simulink model "FlightSim"  (R2023a)
settings: Solver=VariableStepAuto  StartTime=0.0  StopTime=10.0  RelTol=1e-3
model workspace (MAT data in the model file):
  polyCoefficient = [1 1 1]
values from neighbouring files (symbols this model uses):
  mass = 4    [FlightSimSetup.m]
settings Model: Creator=ericyang  LastModifiedBy=ericyang
settings DataIOCC: ExternalInput=[t,u]

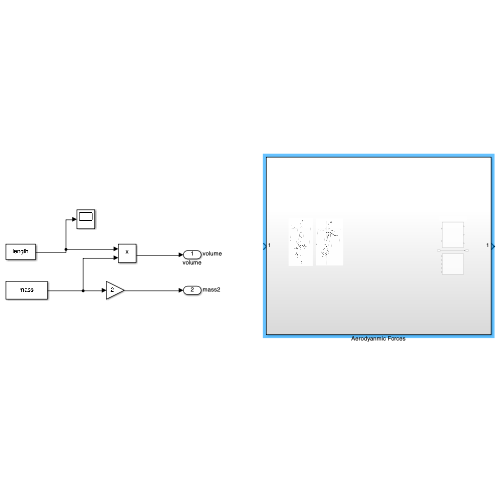
[thumbnail: Simulink's stored preview of the top-level diagram]
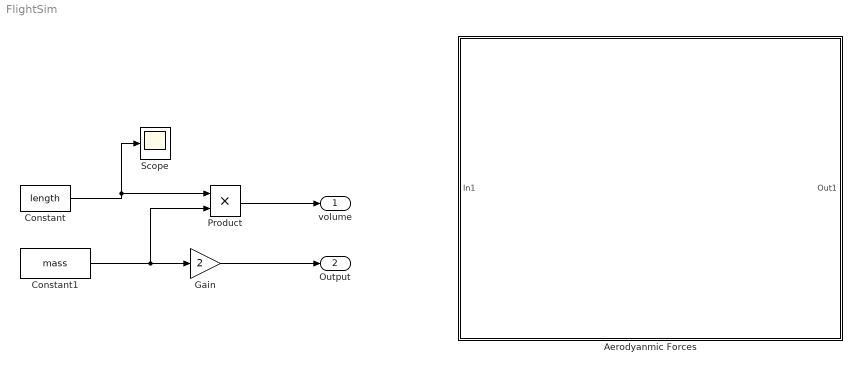
== system FlightSim ==
  Aerodyanmic Forces : Subsystem
  Constant : Constant  Value=length
  Constant1 : Constant  Value=mass
  Gain : Gain  Gain=2
  Product : Product
  Scope : Scope
  volume : Outport  SignalName=volume
  Output : Outport  Port=2  SignalName=mass2
  wires:
  Constant/1 -> Product/1, Scope/1
  Constant1/1 -> Gain/1, Product/2
  Product/1 -> volume/1
  Gain/1 -> Output/1

== system FlightSim/Aerodyanmic Forces ==
  note: calculates the total N and Center of Pressure shown in the diagram based on contriutions from each rocket part, and from those also calculates pitch
  In1 : Inport
  Canard Roll Calc : Subsystem
  Normal Force and Pitch Moment Calc : Subsystem
  Out1 : Outport
  wires:
  In1/1 -> Out1/1

== system FlightSim/Aerodyanmic Forces/Canard Roll Calc ==
  radialMACPosition : Inport
  bodyDiameter : Inport  Port=2
  CNa : Inport  Port=3
  numFins : Inport  Port=4
  rollAngle : Inport  Port=5
  RollForcingCoefficient : Subsystem
  RollForcingCoefficient1 : Subsystem
  wires:
  radialMACPosition/1 -> RollForcingCoefficient/1(radialMACPosition)
  bodyDiameter/1 -> RollForcingCoefficient/2(bodyDiameter)
  CNa/1 -> RollForcingCoefficient/3(CNa)
  numFins/1 -> RollForcingCoefficient/4(numFins)
  rollAngle/1 -> RollForcingCoefficient/5(rollAngle)

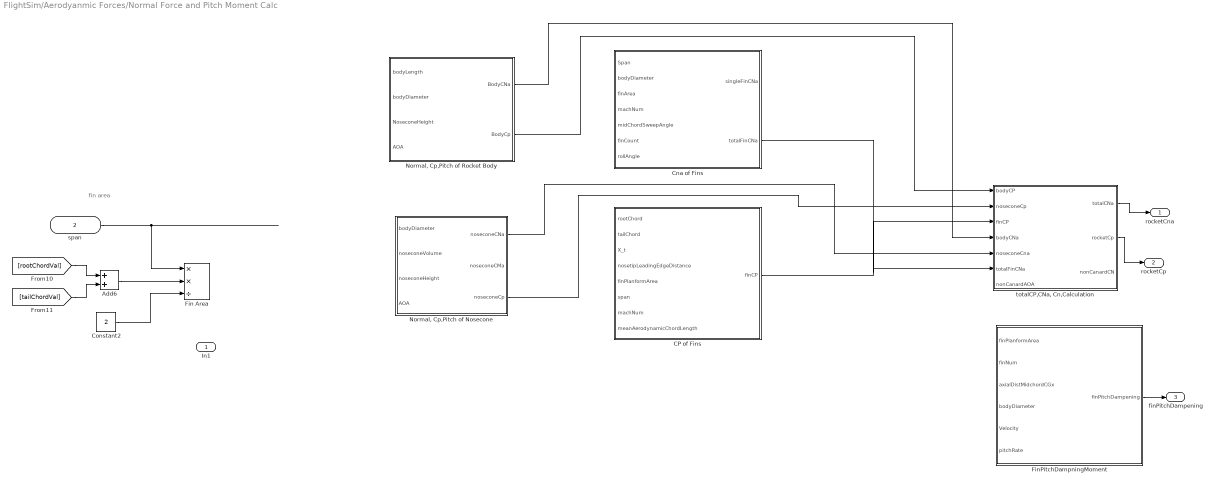
== system FlightSim/Aerodyanmic Forces/Normal Force and Pitch Moment Calc ==
  note: fin area
  In1 : Inport
  span : Inport  Port=2
  Add6 : Sum
  CP of Fins : Subsystem
  Cna of Fins : Subsystem
  Constant2 : Constant  Value=2
  Fin Area : Product  Inputs=**/
  FinPitchDampningMoment : Subsystem
  "Normal, Cp,Pitch of Nosecone" : Subsystem
  "Normal, Cp,Pitch of Rocket Body" : Subsystem
  "totalCP,CNa, Cn,Calculation" : Subsystem
  rocketCna : Outport
  rocketCp : Outport  Port=2
  finPitchDampening : Outport  Port=3
  wires:
  Add6/1 -> Fin Area/2
  span/1 -> Fin Area/1
  [tailChordVal] -> Add6/2
  [rootChordVal] -> Add6/1
  Constant2/1 -> Fin Area/3
  "Normal, Cp,Pitch of Rocket Body"/1(BodyCNa) -> "totalCP,CNa, Cn,Calculation"/4(bodyCNa)
  "Normal, Cp,Pitch of Rocket Body"/2(BodyCp) -> "totalCP,CNa, Cn,Calculation"/1(bodyCP)
  Cna of Fins/2(totalFinCNa) -> "totalCP,CNa, Cn,Calculation"/6(totalFinCNa)
  CP of Fins/1(finCP) -> "totalCP,CNa, Cn,Calculation"/3(finCP)
  "Normal, Cp,Pitch of Nosecone"/3(noseconeCp) -> "totalCP,CNa, Cn,Calculation"/2(noseconeCp)
  "Normal, Cp,Pitch of Nosecone"/1(noseconeCNa) -> "totalCP,CNa, Cn,Calculation"/5(noseconeCna)
  "totalCP,CNa, Cn,Calculation"/1(totalCNa) -> rocketCna/1
  "totalCP,CNa, Cn,Calculation"/2(rocketCp) -> rocketCp/1
  FinPitchDampningMoment/1(finPitchDampening) -> finPitchDampening/1

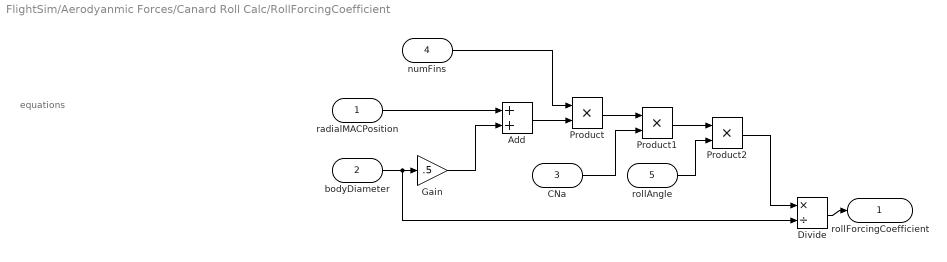
== system FlightSim/Aerodyanmic Forces/Canard Roll Calc/RollForcingCoefficient ==
  note: equations
  radialMACPosition : Inport
  bodyDiameter : Inport  Port=2
  CNa : Inport  Port=3
  numFins : Inport  Port=4
  rollAngle : Inport  Port=5
  Add : Sum
  Divide : Product  Inputs=*/
  Gain : Gain  Gain=.5
  Product : Product
  Product1 : Product
  Product2 : Product
  rollForcingCoefficient : Outport
  wires:
  radialMACPosition/1 -> Add/1
  bodyDiameter/1 -> Divide/2, Gain/1
  rollAngle/1 -> Product2/2
  CNa/1 -> Product1/2
  Divide/1 -> rollForcingCoefficient/1
  Product2/1 -> Divide/1
  Product1/1 -> Product2/1
  Gain/1 -> Add/2
  Product/1 -> Product1/1
  numFins/1 -> Product/1
  Add/1 -> Product/2

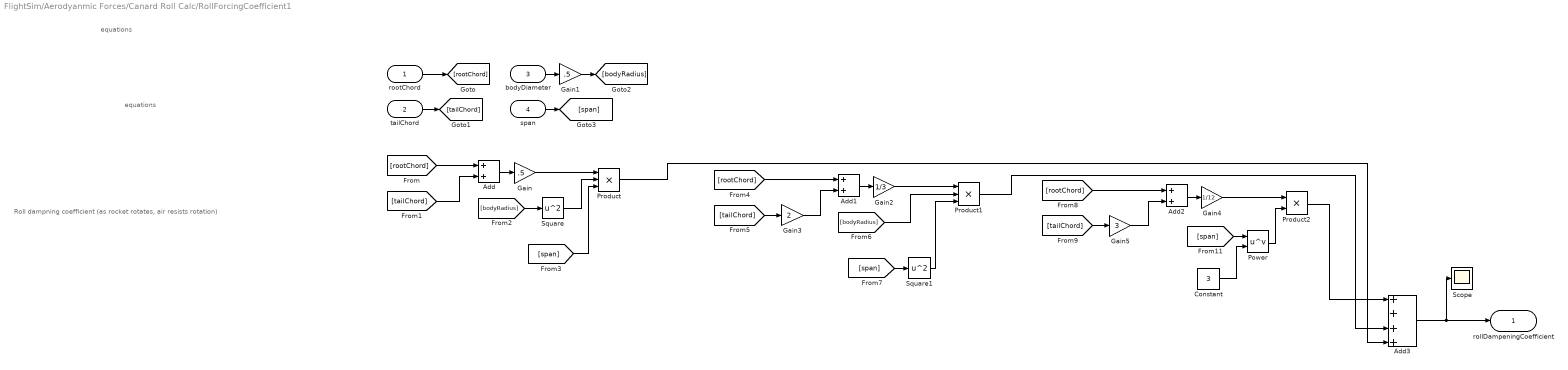
== system FlightSim/Aerodyanmic Forces/Canard Roll Calc/RollForcingCoefficient1 ==
  note: Roll dampning coefficient (as rocket rotates, air resists rotation)
  note: equations
  note: equations
  rootChord : Inport
  tailChord : Inport  Port=2
  bodyDiameter : Inport  Port=3
  span : Inport  Port=4
  Add : Sum
  Add1 : Sum
  Add2 : Sum
  Add3 : Sum  Inputs=++++
  Constant : Constant  Value=3
  Gain : Gain  Gain=.5
  Gain1 : Gain  Gain=.5
  Gain2 : Gain  Gain=1/3
  Gain3 : Gain  Gain=2
  Gain4 : Gain  Gain=1/12
  Gain5 : Gain  Gain=3
  Power : Math  Operator=pow
  Product : Product  Inputs=3
  Product1 : Product  Inputs=3
  Product2 : Product
  Scope : Scope
  Square : Math  Operator=square
  Square1 : Math  Operator=square
  rollDampeningCoefficient : Outport
  wires:
  Add/1 -> Gain/1
  rootChord/1 -> [rootChord]
  tailChord/1 -> [tailChord]
  bodyDiameter/1 -> Gain1/1
  span/1 -> [span]
  [rootChord] -> Add/1
  [tailChord] -> Add/2
  Gain/1 -> Product/1
  Gain1/1 -> [bodyRadius]
  [bodyRadius] -> Square/1
  Square/1 -> Product/2
  [span] -> Product/3
  [tailChord] -> Gain3/1
  [rootChord] -> Add1/1
  Add1/1 -> Gain2/1
  Gain2/1 -> Product1/1
  Gain3/1 -> Add1/2
  [span] -> Square1/1
  Square1/1 -> Product1/3
  [bodyRadius] -> Product1/2
  [span] -> Power/1
  [tailChord] -> Gain5/1
  Gain5/1 -> Add2/2
  [rootChord] -> Add2/1
  Add2/1 -> Gain4/1
  Gain4/1 -> Product2/1
  Constant/1 -> Power/2
  Power/1 -> Product2/2
  Product2/1 -> Add3/1
  Product1/1 -> Add3/3
  Product/1 -> Add3/4
  Add3/1 -> Scope/1, rollDampeningCoefficient/1

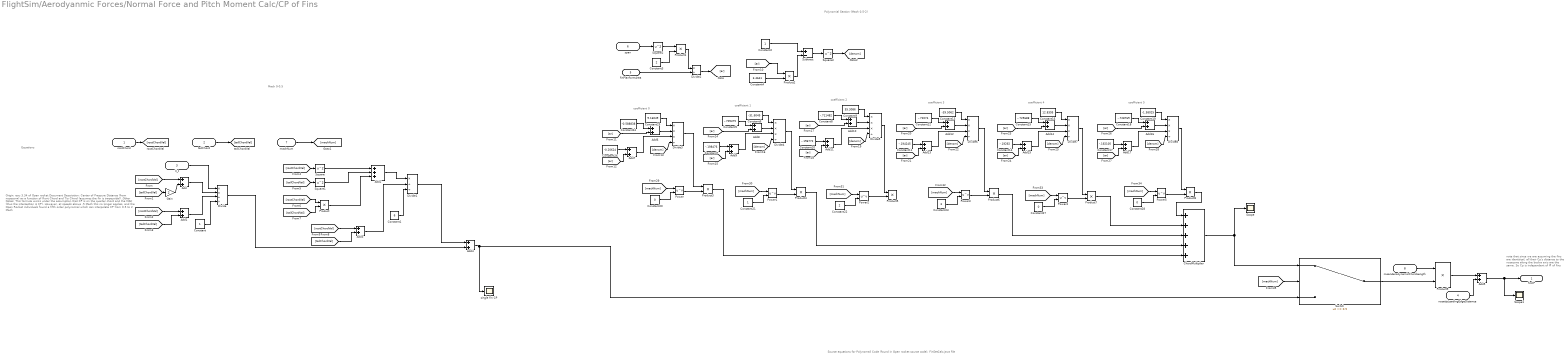
== system FlightSim/Aerodyanmic Forces/Normal Force and Pitch Moment Calc/CP of Fins ==
  note: note that since we are assuming the fins are identitical, all their Cp's distance to the nosecone along the bodya axis are the same. So Cp is independent of # of fins
  note: Mach 0-0.5
  note: Source equations for Polynomail Code (found in Open rocket source code), FinSetCalc.java file
  note: Polynomial Section (Mach 0.5-2)
  note: coefficient 0
  note: Equations
  note: Origin: equ 3.34  of Open rocket Document
      |
      | Description: Center of Pressure Distance (from nosecone)
      | as a function of Root Chord and Tip Chord (assumes the fin is trapezoidal).
      |
      | Other Notes: This formula works under the assumption that CP is on the quarter chord
      | and the MAC (thus the intersection is CP). However, at speeds above .5 Mach this no longer applies, and the Open Rocket individuals found a fifth order polynomial which can interpolate CP from 0.5 to 2 Mach
  note: coefficient 1
  note: coefficient 2
  note: coefficient 3
  note: coefficient 4
  note: coefficient 5
  rootChord : Inport
  tailChord : Inport  Port=2
  X_t : Inport  Port=3
  nosetipLeadingEdgeDistance : Inport  Port=4
  finPlanformArea : Inport  Port=5
  span : Inport  Port=6
  machNum : Inport  Port=7
  meanAerodynamicChordLength : Inport  Port=8
  Add{,1,3..17} (17 alike) : Sum
  Add2 : Sum  Inputs=+++
  ChordMultiplier : Sum  Inputs=+++++
  Constant : Constant
  Constant1 : Constant  Value=6
  Constant10 : Constant  Value=-.196772
  Constant11 : Constant  Value=-.194245
  Constant12 : Constant  Value=-.72074
  Constant13 : Constant  Value=-39.5062
  Constant14 : Constant  Value=-.19292
  Constant15 : Constant  Value=-.725688
  Constant16 : Constant  Value=12.8395
  Constant17 : Constant  Value=-.192105
  Constant18 : Constant  Value=-.728769
  Constant19 : Constant  Value=-1.58025
  Constant2 : Constant
  Constant20 : Constant  Value=0
  Constant21 : Constant
  Constant22 : Constant  Value=2
  Constant23 : Constant  Value=3
  Constant24 : Constant  Value=-0.588838
  Constant25 : Constant  Value=9.16049
  Constant26 : Constant  Value=-0.20624
  Constant27 : Constant  Value=0
  Constant28 : Constant  Value=0
  Constant3 : Constant  Value=2
  Constant4 : Constant  Value=3.4641
  Constant5 : Constant  Value=-.705375
  Constant6 : Constant  Value=-31.6049
  Constant7 : Constant  Value=-.198476
  Constant8 : Constant  Value=-.711482
  Constant9 : Constant  Value=55.3086
  Divide : Product  Inputs=**//
  Divide1 : Product  Inputs=*//
  Divide2 : Product  Inputs=*/
  Divide{3..8} (6 alike) : Product  Inputs=***/
  Gain : Gain  Gain=2
  Power{,1..5} (6 alike) : Math  Operator=pow
  Product{,1..9} (10 alike) : Product
  Scope : Scope
  Scope1 : Scope
  Square{,1..3} (4 alike) : Math  Operator=square
  Subtract : Sum  Inputs=+-
  Switch : Switch  Threshold=0.5  SaturateOnIntegerOverflow=off  InputSameDT=off
  single fin CP : Scope
  finCP : Outport
  wires:
  rootChord/1 -> [rootChordVal]
  tailChord/1 -> [tailChordVal]
  [rootChordVal] -> Add/1
  [tailChordVal] -> Gain/1
  Gain/1 -> Add/2
  [rootChordVal] -> Add1/1
  [tailChordVal] -> Add1/2
  Add/1 -> Divide/2
  Add1/1 -> Divide/3
  Constant/1 -> Divide/4
  X_t/1 -> Divide/1
  [rootChordVal] -> Square/1
  Square/1 -> Add2/1
  [tailChordVal] -> Square1/1
  Square1/1 -> Add2/2
  [rootChordVal] -> Product/1
  [tailChordVal] -> Product/2
  Product/1 -> Add2/3
  Add2/1 -> Divide1/1
  [tailChordVal] -> Add3/2
  [rootChordVal] -> Add3/1
  Add3/1 -> Divide1/2
  Constant1/1 -> Divide1/3
  Divide/1 -> Add4/2
  Divide1/1 -> Add4/1
  Add4/1 -> Switch/3, single fin CP/1
  Constant3/1 -> Product1/2
  Square2/1 -> Product1/1
  Product1/1 -> Divide2/1
  finPlanformArea/1 -> Divide2/2
  span/1 -> Square2/1
  Divide2/1 -> [ar]
  machNum/1 -> [machNum]
  Constant4/1 -> Product2/2
  [ar] -> Product2/1
  Constant2/1 -> Subtract/1
  Product2/1 -> Subtract/2
  Subtract/1 -> Square3/1
  Square3/1 -> [denom]
  Constant25/1 -> Divide3/1
  Constant24/1 -> Add6/1
  [ar] -> Add6/2
  Constant26/1 -> Add7/1
  [ar] -> Add7/2
  Add7/1 -> Divide3/3
  Add6/1 -> Divide3/2
  [denom] -> Divide3/4
  [ar] -> Add9/2
  Constant7/1 -> Add9/1
  Add8/1 -> Divide4/2
  Constant6/1 -> Divide4/1
  Constant5/1 -> Add8/1
  [denom] -> Divide4/4
  Add9/1 -> Divide4/3
  [ar] -> Add8/2
  Add11/1 -> Divide5/3
  Constant10/1 -> Add11/1
  [denom] -> Divide5/4
  Add10/1 -> Divide5/2
  [ar] -> Add10/2
  [ar] -> Add11/2
  Constant8/1 -> Add10/1
  Constant9/1 -> Divide5/1
  [ar] -> Add12/2
  [denom] -> Divide6/4
  Constant11/1 -> Add13/1
  [ar] -> Add13/2
  Constant12/1 -> Add12/1
  Constant13/1 -> Divide6/1
  Add13/1 -> Divide6/3
  Add12/1 -> Divide6/2
  [ar] -> Add14/2
  Constant14/1 -> Add15/1
  Constant15/1 -> Add14/1
  [denom] -> Divide7/4
  Add14/1 -> Divide7/2
  Add15/1 -> Divide7/3
  [ar] -> Add15/2
  Constant16/1 -> Divide7/1
  Constant19/1 -> Divide8/1
  [ar] -> Add16/2
  Add17/1 -> Divide8/3
  [ar] -> Add17/2
  [denom] -> Divide8/4
  Add16/1 -> Divide8/2
  Constant17/1 -> Add17/1
  Constant18/1 -> Add16/1
  Divide3/1 -> Product3/1
  [machNum] -> Power/1
  Constant20/1 -> Power/2
  Power/1 -> Product3/2
  [machNum] -> Power1/1
  Constant21/1 -> Power1/2
  Power1/1 -> Product4/2
  Divide4/1 -> Product4/1
  [machNum] -> Power2/1
  Constant22/1 -> Power2/2
  Power2/1 -> Product5/2
  Divide5/1 -> Product5/1
  [machNum] -> Power3/1
  Constant23/1 -> Power3/2
  Power3/1 -> Product6/2
  Divide6/1 -> Product6/1
  [machNum] -> Power4/1
  Constant27/1 -> Power4/2
  Power4/1 -> Product7/2
  Divide7/1 -> Product7/1
  [machNum] -> Power5/1
  Constant28/1 -> Power5/2
  Power5/1 -> Product8/2
  Divide8/1 -> Product8/1
  Product8/1 -> ChordMultiplier/1
  Product7/1 -> ChordMultiplier/2
  Product3/1 -> ChordMultiplier/5
  Product4/1 -> ChordMultiplier/4
  Product6/1 -> ChordMultiplier/3
  [machNum] -> Switch/2
  ChordMultiplier/1 -> Switch/1, Scope/1
  meanAerodynamicChordLength/1 -> Product9/1
  Switch/1 -> Product9/2
  Product9/1 -> Add5/1
  nosetipLeadingEdgeDistance/1 -> Add5/2
  Add5/1 -> Scope1/1, finCP/1

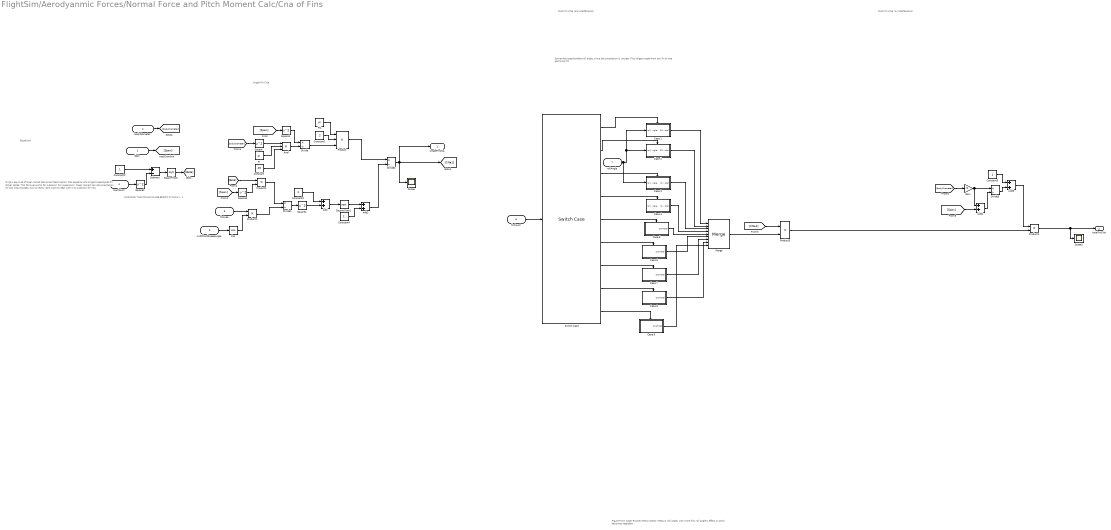
== system FlightSim/Aerodyanmic Forces/Normal Force and Pitch Moment Calc/Cna of Fins ==
  note: WARNING: THIS COULD CAUSE ERROR IF MACH > 1
  note: Origin: equ 3.40  of Open rocket Document
      |
      | Description: CNa equation of a single trapezopidal fin
      |
      | Other Notes: This formual works for subsonic. For supersonic, Open rockert has documentation on how CNa changes, but currently dont want to deal with it so subsonic for now
  note: Equations
  note: Single Fin CNa
  note: Multi Fin CNa (w/ interference)
  note: Somewhat questionable roll angle, since documentation is unclear if its largest angle from any fin or one particular fin
  note: FIgure From Open Rocket Thesis
      |
      | Notes: Theta is roll angle, with more fins roll angle's effect on pitch becomes negligble
  note: Multi Fin CNa (pre interference)
  Span : Inport
  bodyDiameter : Inport  Port=2
  finArea : Inport  Port=3
  machNum : Inport  Port=4
  midChordSweepAngle : Inport  Port=5
  finCount : Inport  Port=6
  rollAngle : Inport  Port=7
  Add{,1..3} (4 alike) : Sum
  Aref : Product  Inputs=3
  Case 1 : Subsystem  TreatAsAtomicUnit=on
  Case 2 : Subsystem  TreatAsAtomicUnit=on
  Case 3 : Subsystem  TreatAsAtomicUnit=on
  Case 4 : Subsystem  TreatAsAtomicUnit=on
  Case 5 : Subsystem  TreatAsAtomicUnit=on
  Case 6 : Subsystem  TreatAsAtomicUnit=on
  Case 7 : Subsystem  TreatAsAtomicUnit=on
  Case 8 : Subsystem  TreatAsAtomicUnit=on
  Case 9 : Subsystem  TreatAsAtomicUnit=on
  Constant : Constant  Value=.25
  Constant1 : Constant  Value=2
  Constant{2..5} (4 alike) : Constant
  Cos : Trigonometry  Operator=cos
  Divide : Product  Inputs=*/
  Divide1 : Product  Inputs=*/
  Divide2 : Product  Inputs=*/
  Divide3 : Product  Inputs=*/  RndMeth=Zero  SaturateOnIntegerOverflow=on
  Gain : Gain  Gain=.5
  Merge : Merge  Inputs=9
  Pi : Constant  Value=pi  OutDataTypeStr=Inherit: Inherit via back propagation
  Pi1 : Constant  Value=pi  OutDataTypeStr=Inherit: Inherit via back propagation
  Product : Product  Inputs=3
  Product{1..4} (4 alike) : Product
  Scope : Scope
  Scope1 : Scope
  Square{,1..4} (5 alike) : Math  Operator=square
  Square Root : Sqrt
  Square Root1 : Sqrt
  Subtract : Sum  Inputs=+-
  Switch Case : SwitchCase  CaseConditions={1,2,3,4,5,6,7,8}
  singleFinCNa : Outport
  totalFinCNa : Outport  Port=2
  wires:
  Span/1 -> [Span]
  Constant/1 -> Aref/3
  bodyDiameter/1 -> [bodyDiameter]
  Square/1 -> Aref/1
  Pi/1 -> Aref/2
  [Span] -> Square1/1
  Square1/1 -> Divide/1
  Aref/1 -> Divide/2
  Pi1/1 -> Product/1
  Constant1/1 -> Product/2
  Divide/1 -> Product/3
  Constant2/1 -> Subtract/1
  machNum/1 -> Square2/1
  Square2/1 -> Subtract/2
  Subtract/1 -> Square Root/1
  Square Root/1 -> [Beta]
  [Span] -> Square3/1
  [Beta] -> Product1/1
  Square3/1 -> Product1/2
  Product1/1 -> Divide1/1
  finArea/1 -> Product2/1
  midChordSweepAngle/1 -> Cos/1
  Cos/1 -> Product2/2
  Product2/1 -> Divide1/2
  Divide1/1 -> Square4/1
  Constant3/1 -> Add/1
  Square4/1 -> Add/2
  Add/1 -> Square Root1/1
  Constant4/1 -> Add1/2
  Square Root1/1 -> Add1/1
  Product/1 -> Divide2/1
  Add1/1 -> Divide2/2
  Divide2/1 -> [CNa1], Scope/1, singleFinCNa/1
  finCount/1 -> Switch Case/1
  Switch Case/1 -> Case 1/Action
  rollAngle/1 -> Case 3/1(rollAngle), Case 1/1(rollAngle), Case 2/1(rollAngle)
  Switch Case/2 -> Case 2/Action
  Switch Case/3 -> Case 3/Action
  Switch Case/4 -> Case 4/Action
  Switch Case/5 -> Case 5/Action
  Switch Case/9 -> Case 9/Action
  Switch Case/8 -> Case 8/Action
  Switch Case/7 -> Case 7/Action
  Switch Case/6 -> Case 6/Action
  Case 1/1(CNaTotal) -> Merge/1
  Case 2/1(CNaTotal) -> Merge/2
  Case 3/1(CnaTotal) -> Merge/3
  Case 4/1(CnaTotal) -> Merge/4
  Case 5/1(CnaTotal) -> Merge/5
  Case 6/1(CnaTotal) -> Merge/6
  Case 7/1(CnaTotal) -> Merge/7
  Case 8/1(CnaTotal) -> Merge/8
  Case 9/1(CnaTotal) -> Merge/9
  [CNa1] -> Product3/1
  Merge/1 -> Product3/2
  [bodyDiameter] -> Square/1
  [bodyDiameter] -> Gain/1
  Gain/1 -> Add2/1, Divide3/1
  [Span] -> Add2/2
  Divide3/1 -> Add3/2
  Add2/1 -> Divide3/2
  Constant5/1 -> Add3/1
  Add3/1 -> Product4/1
  Product3/1 -> Product4/2
  Product4/1 -> Scope1/1, totalFinCNa/1

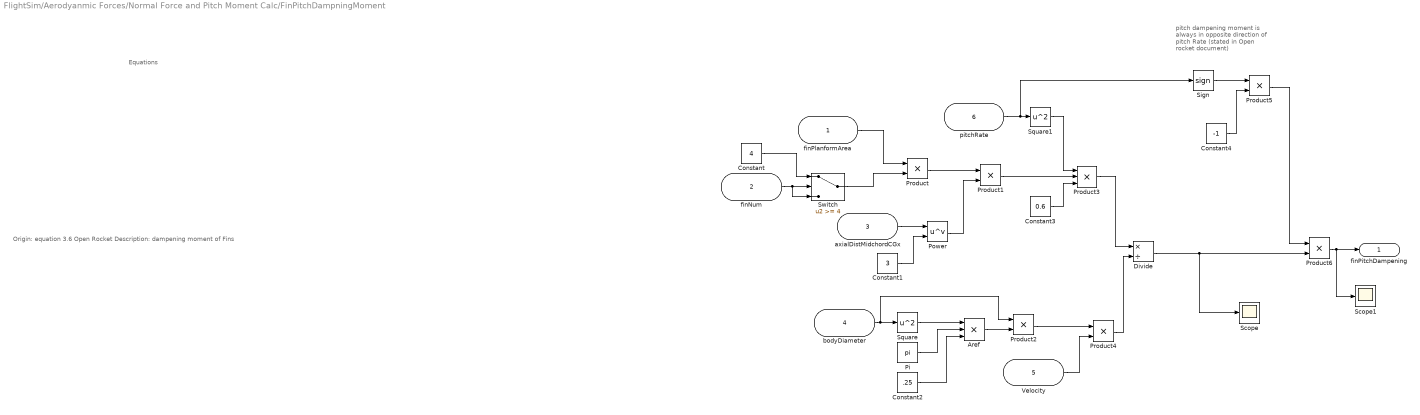
== system FlightSim/Aerodyanmic Forces/Normal Force and Pitch Moment Calc/FinPitchDampningMoment ==
  note: pitch dampening moment is always in opposite direction of pitch Rate (stated in Open rocket document)
  note: Origin: equation 3.6 Open Rocket
      |
      | Description: dampening moment of Fins
  note: Equations
  finPlanformArea : Inport
  finNum : Inport  Port=2
  axialDistMidchordCGx : Inport  Port=3
  bodyDiameter : Inport  Port=4
  Velocity : Inport  Port=5
  pitchRate : Inport  Port=6
  Aref : Product  Inputs=3
  Constant : Constant  Value=4
  Constant1 : Constant  Value=3
  Constant2 : Constant  Value=.25
  Constant3 : Constant  Value=0.6
  Constant4 : Constant  Value=-1
  Divide : Product  Inputs=*/
  Pi : Constant  Value=pi  OutDataTypeStr=Inherit: Inherit via back propagation
  Power : Math  Operator=pow
  Product{,1..2,4..6} (6 alike) : Product
  Product3 : Product  Inputs=3
  Scope : Scope
  Scope1 : Scope
  Sign : Signum
  Square : Math  Operator=square
  Square1 : Math  Operator=square
  Switch : Switch  Threshold=4  SaturateOnIntegerOverflow=off  InputSameDT=off
  finPitchDampening : Outport
  wires:
  finNum/1 -> Switch/3, Switch/2
  Constant/1 -> Switch/1
  Switch/1 -> Product/2
  finPlanformArea/1 -> Product/1
  axialDistMidchordCGx/1 -> Power/1
  Constant1/1 -> Power/2
  Power/1 -> Product1/2
  Product/1 -> Product1/1
  Constant2/1 -> Aref/3
  bodyDiameter/1 -> Product2/1, Square/1
  Square/1 -> Aref/1
  Pi/1 -> Aref/2
  Aref/1 -> Product2/2
  pitchRate/1 -> Sign/1, Square1/1
  Square1/1 -> Product3/1
  Product1/1 -> Product3/2
  Constant3/1 -> Product3/3
  Product2/1 -> Product4/1
  Velocity/1 -> Product4/2
  Product3/1 -> Divide/1
  Product4/1 -> Divide/2
  Divide/1 -> Product6/2, Scope/1
  Constant4/1 -> Product5/2
  Sign/1 -> Product5/1
  Product5/1 -> Product6/1
  Product6/1 -> Scope1/1, finPitchDampening/1

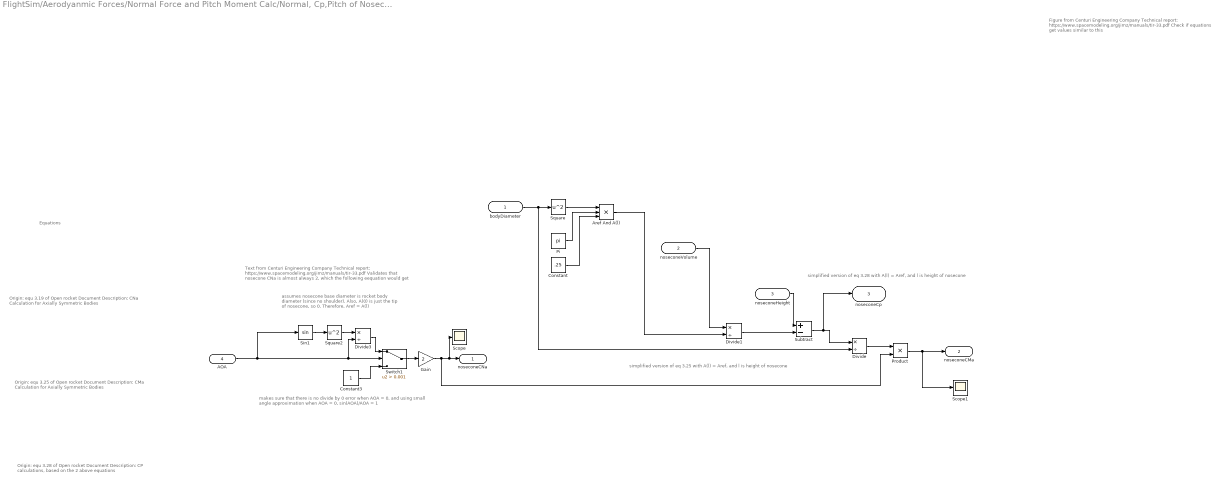
== system FlightSim/Aerodyanmic Forces/Normal Force and Pitch Moment Calc/Normal, Cp,Pitch of Nosecone ==
  note: simplified version of eq 3.25 with A(l) = Aref, and l is height of nosecone
  note: assumes nosecone base diameter is rocket body diameter (since no shoulder). Also, A(0) is just the tip of nosecone, so 0. Therefore, Aref = A(l)
  note: Equations
  note: Origin: equ 3.19  of Open rocket Document
      |
      | Description: CNa Calculation for Axially Symmetric Bodies
  note: Origin: equ 3.25  of Open rocket Document
      |
      | Description: CMa Calculation for Axially Symmetric Bodies
  note: Origin: equ 3.28  of Open rocket Document
      |
      | Description: CP calculations, based on the 2 above equations
  note: makes sure that there is no divide by 0 error when AOA = 0,
      | and using small angle approximation when AOA = 0, sin(AOA)/AOA = 1
  note: simplified version of eq 3.28 with A(l) = Aref, and l is height of nosecone
  note: Text from Centuri Engineering Company Technical report: https://www.spacemodeling.org/jimz/manuals/tir-33.pdf
      | Validates that nosecone CNa is almost always 2, which the following eequation would get
  note: Figure from Centuri Engineering Company Technical report: https://www.spacemodeling.org/jimz/manuals/tir-33.pdf
      | Check if equations get values similar to this
  bodyDiameter : Inport
  noseconeVolume : Inport  Port=2
  noseconeHeight : Inport  Port=3
  AOA : Inport  Port=4
  Aref And A(l) : Product  Inputs=3
  Constant : Constant  Value=.25
  Constant3 : Constant
  Divide : Product  Inputs=*/
  Divide1 : Product  Inputs=*/
  Divide3 : Product  Inputs=*/
  Gain : Gain  Gain=2
  Pi : Constant  Value=pi  OutDataTypeStr=Inherit: Inherit via back propagation
  Product : Product
  Scope : Scope
  Scope1 : Scope
  Sin1 : Trigonometry
  Square : Math  Operator=square
  Square2 : Math  Operator=square
  Subtract : Sum  Inputs=+-
  Switch1 : Switch  Criteria=u2 > Threshold  Threshold=0.001  SaturateOnIntegerOverflow=off  InputSameDT=off
  noseconeCNa : Outport
  noseconeCMa : Outport  Port=2
  noseconeCp : Outport  Port=3
  wires:
  Square/1 -> Aref And A(l)/1
  Pi/1 -> Aref And A(l)/2
  Constant/1 -> Aref And A(l)/3
  Square2/1 -> Divide3/1
  AOA/1 -> Sin1/1, Divide3/2, Switch1/2
  Divide3/1 -> Switch1/1
  Constant3/1 -> Switch1/3
  Sin1/1 -> Square2/1
  Gain/1 -> Product/2, Scope/1, noseconeCNa/1
  noseconeVolume/1 -> Divide1/1
  noseconeHeight/1 -> Subtract/1
  Divide1/1 -> Subtract/2
  Subtract/1 -> noseconeCp/1, Divide/1
  Divide/1 -> Product/1
  Switch1/1 -> Gain/1
  Product/1 -> Scope1/1, noseconeCMa/1
  Aref And A(l)/1 -> Divide1/2
  bodyDiameter/1 -> Divide/2, Square/1

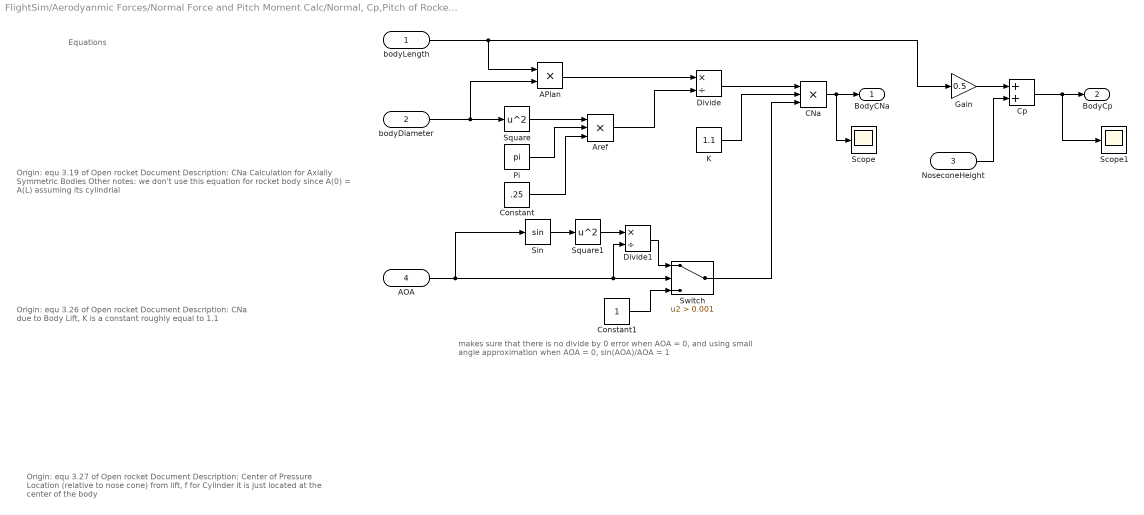
== system FlightSim/Aerodyanmic Forces/Normal Force and Pitch Moment Calc/Normal, Cp,Pitch of Rocket Body ==
  note: makes sure that there is no divide by 0 error when AOA = 0,
      | and using small angle approximation when AOA = 0, sin(AOA)/AOA = 1
  note: Equations
  note: Origin: equ 3.19  of Open rocket Document
      |
      | Description: CNa Calculation for Axially Symmetric Bodies
      |
      | Other notes: we don't use this equation for rocket body since A(0) = A(L) assuming
      | its cylindrial
  note: Origin: equ 3.26  of Open rocket Document
      |
      | Description: CNa due to Body Lift, K is a constant roughly
      | equal to 1.1
  note: Origin: equ 3.27 of Open rocket Document
      |
      | Description: Center of Pressure Location (relative to nose cone) from lift, f
      | for Cylinder it is just located at the center of the body
  bodyLength : Inport
  bodyDiameter : Inport  Port=2
  NoseconeHeight : Inport  Port=3
  AOA : Inport  Port=4
  APlan : Product
  Aref : Product  Inputs=3
  CNa : Product  Inputs=3
  Constant : Constant  Value=.25
  Constant1 : Constant
  Cp : Sum
  Divide : Product  Inputs=*/
  Divide1 : Product  Inputs=*/
  Gain : Gain  Gain=0.5
  K : Constant  Value=1.1
  Pi : Constant  Value=pi  OutDataTypeStr=Inherit: Inherit via back propagation
  Scope : Scope
  Scope1 : Scope
  Sin : Trigonometry
  Square : Math  Operator=square
  Square1 : Math  Operator=square
  Switch : Switch  Criteria=u2 > Threshold  Threshold=0.001  SaturateOnIntegerOverflow=off  InputSameDT=off
  BodyCNa : Outport
  BodyCp : Outport  Port=2
  wires:
  bodyLength/1 -> Gain/1, APlan/1
  bodyDiameter/1 -> APlan/2, Square/1
  Constant/1 -> Aref/3
  Pi/1 -> Aref/2
  Square/1 -> Aref/1
  APlan/1 -> Divide/1
  Aref/1 -> Divide/2
  AOA/1 -> Sin/1, Divide1/2, Switch/2
  Sin/1 -> Square1/1
  Divide/1 -> CNa/1
  K/1 -> CNa/2
  Gain/1 -> Cp/1
  NoseconeHeight/1 -> Cp/2
  CNa/1 -> Scope/1, BodyCNa/1
  Cp/1 -> Scope1/1, BodyCp/1
  Switch/1 -> CNa/3
  Square1/1 -> Divide1/1
  Divide1/1 -> Switch/1
  Constant1/1 -> Switch/3

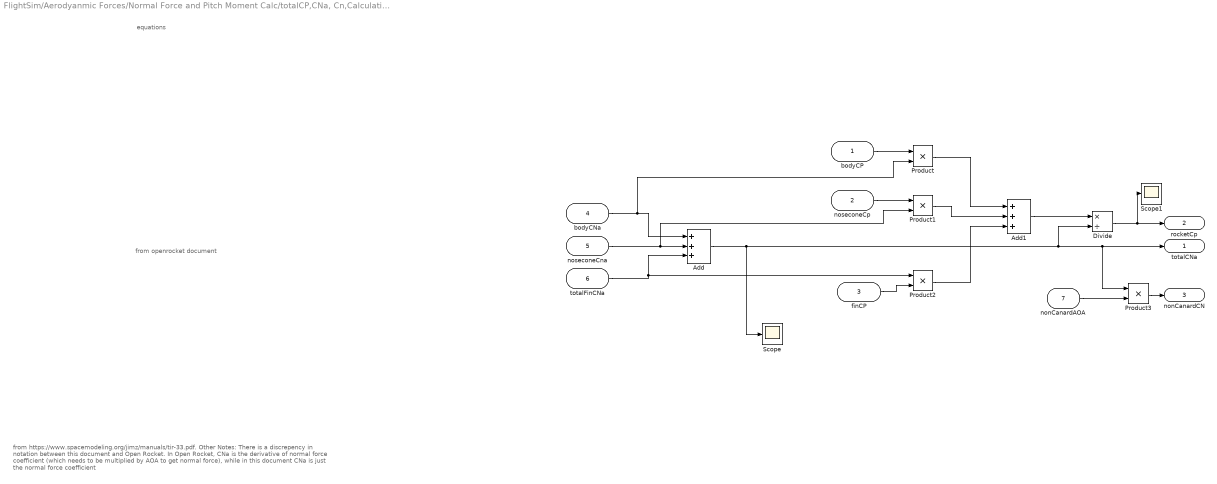
== system FlightSim/Aerodyanmic Forces/Normal Force and Pitch Moment Calc/totalCP,CNa, Cn,Calculation ==
  note: from openrocket document
  note: equations
  note: from https://www.spacemodeling.org/jimz/manuals/tir-33.pdf.
      |
      | Other Notes: There is a discrepency in notation between this document and Open Rocket. In Open Rocket, CNa is the derivative of normal force coefficient (which needs to be multiplied by AOA to get normal force), while in this document CNa is just the normal force coefficient
  bodyCP : Inport
  noseconeCp : Inport  Port=2
  finCP : Inport  Port=3
  bodyCNa : Inport  Port=4
  noseconeCna : Inport  Port=5
  totalFinCNa : Inport  Port=6
  nonCanardAOA : Inport  Port=7
  Add : Sum  Inputs=+++
  Add1 : Sum  Inputs=+++
  Divide : Product  Inputs=*/
  Product{,1..3} (4 alike) : Product
  Scope : Scope
  Scope1 : Scope
  totalCNa : Outport
  rocketCp : Outport  Port=2
  nonCanardCN : Outport  Port=3
  wires:
  totalFinCNa/1 -> Product2/1, Add/3
  noseconeCna/1 -> Product1/2, Add/2
  bodyCNa/1 -> Product/2, Add/1
  Add/1 -> Product3/1, totalCNa/1, Divide/2, Scope/1
  bodyCP/1 -> Product/1
  noseconeCp/1 -> Product1/1
  finCP/1 -> Product2/2
  Product/1 -> Add1/1
  Product1/1 -> Add1/2
  Product2/1 -> Add1/3
  Add1/1 -> Divide/1
  Divide/1 -> Scope1/1, rocketCp/1
  nonCanardAOA/1 -> Product3/2
  Product3/1 -> nonCanardCN/1

== system FlightSim/Aerodyanmic Forces/Normal Force and Pitch Moment Calc/Cna of Fins/Case 1 ==
  rollAngle : Inport
  Action Port : ActionPort  ActionPortLabel=case [ 1 ]:
  Sin : Trigonometry
  Square5 : Math  Operator=square
  CNaTotal : Outport
  wires:
  Sin/1 -> Square5/1
  rollAngle/1 -> Sin/1
  Square5/1 -> CNaTotal/1

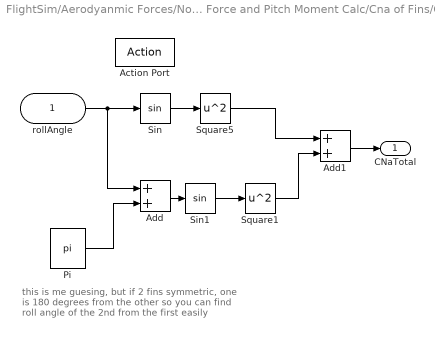
== system FlightSim/Aerodyanmic Forces/Normal Force and Pitch Moment Calc/Cna of Fins/Case 2 ==
  note: this is me guesing, but if 2 fins symmetric, one is 180 degrees from the other so you can find roll angle of the 2nd from the first easily
  rollAngle : Inport
  Action Port : ActionPort  ActionPortLabel=case [ 2 ]:
  Add : Sum
  Add1 : Sum
  Pi : Constant  Value=pi  OutDataTypeStr=Inherit: Inherit via back propagation
  Sin : Trigonometry
  Sin1 : Trigonometry
  Square1 : Math  Operator=square
  Square5 : Math  Operator=square
  CNaTotal : Outport
  wires:
  Add1/1 -> CNaTotal/1
  Sin/1 -> Square5/1
  rollAngle/1 -> Add/1, Sin/1
  Square5/1 -> Add1/1
  Pi/1 -> Add/2
  Sin1/1 -> Square1/1
  Add/1 -> Sin1/1
  Square1/1 -> Add1/2

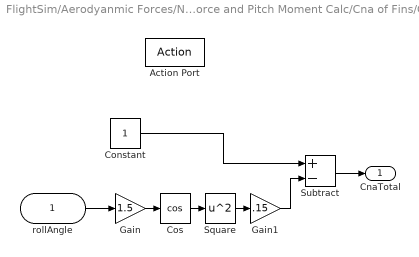
== system FlightSim/Aerodyanmic Forces/Normal Force and Pitch Moment Calc/Cna of Fins/Case 3 ==
  rollAngle : Inport
  Action Port : ActionPort  ActionPortLabel=case [ 3 ]:
  Constant : Constant
  Cos : Trigonometry  Operator=cos
  Gain : Gain  Gain=1.5
  Gain1 : Gain  Gain=.15
  Square : Math  Operator=square
  Subtract : Sum  Inputs=+-
  CnaTotal : Outport
  wires:
  Constant/1 -> Subtract/1
  rollAngle/1 -> Gain/1
  Gain/1 -> Cos/1
  Cos/1 -> Square/1
  Square/1 -> Gain1/1
  Gain1/1 -> Subtract/2
  Subtract/1 -> CnaTotal/1

== system FlightSim/Aerodyanmic Forces/Normal Force and Pitch Moment Calc/Cna of Fins/Case 4 ==
  rollAngle : Inport
  Action Port : ActionPort  ActionPortLabel=case [ 4 ]:
  Constant : Constant
  Cos : Trigonometry
  Gain : Gain  Gain=2
  Gain1 : Gain  Gain=0.06
  Square : Math  Operator=square
  Subtract : Sum  Inputs=+-
  CnaTotal : Outport
  wires:
  Constant/1 -> Subtract/1
  rollAngle/1 -> Gain/1
  Gain/1 -> Cos/1
  Cos/1 -> Square/1
  Square/1 -> Gain1/1
  Gain1/1 -> Subtract/2
  Subtract/1 -> CnaTotal/1

== system FlightSim/Aerodyanmic Forces/Normal Force and Pitch Moment Calc/Cna of Fins/Case 5 ==
  Action Port : ActionPort  ActionPortLabel=case [ 5 ]:
  Constant : Constant  Value=2.37
  CnaTotal : Outport
  wires:
  Constant/1 -> CnaTotal/1

== system FlightSim/Aerodyanmic Forces/Normal Force and Pitch Moment Calc/Cna of Fins/Case 6 ==
  Action Port : ActionPort  ActionPortLabel=case [ 6 ]:
  Constant : Constant  Value=2.74
  CnaTotal : Outport
  wires:
  Constant/1 -> CnaTotal/1

== system FlightSim/Aerodyanmic Forces/Normal Force and Pitch Moment Calc/Cna of Fins/Case 7 ==
  Action Port : ActionPort  ActionPortLabel=case [ 7 ]:
  Constant : Constant  Value=2.99
  CnaTotal : Outport
  wires:
  Constant/1 -> CnaTotal/1

== system FlightSim/Aerodyanmic Forces/Normal Force and Pitch Moment Calc/Cna of Fins/Case 8 ==
  Action Port : ActionPort  ActionPortLabel=case [ 8 ]:
  Constant : Constant  Value=3.24
  CnaTotal : Outport
  wires:
  Constant/1 -> CnaTotal/1

== system FlightSim/Aerodyanmic Forces/Normal Force and Pitch Moment Calc/Cna of Fins/Case 9 ==
  Action Port : ActionPort  ActionPortLabel=default:
  Constant : Constant  Value=2
  CnaTotal : Outport
  wires:
  Constant/1 -> CnaTotal/1
